simulink model "pfb_fir_8192chb_core"  (R2016b)
settings: Solver=ode45  StartTime=0.0  StopTime=10.0  RelTol=1e-3  EnableMultiTasking=on
undefined symbols (not defined in the file or in its folder): pfb_coeff_gen_calc
libraries: xbsIndex_r4 x853, casper_library_delays x48, simulink x2
(part 1 of 11)
settings Model: Creator=zaki  LastModifiedBy=kocz
settings DataIOCC: LimitDataPoints=on  SaveFormat=Array  SignalLoggingSaveFormat=ModelDataLogs
settings OptimizationCC: ExpressionDepthLimit=2147483647  LifeSpan=inf
settings DebuggingCC: UnderspecifiedInitializationDetection=Classic  MergeDetectMultiDrivingBlocksExec=none  SolverPrmCheckMsg=warning  FcnCallInpInsideContextMsg=warning  StateNameClashWarn=warning  SFUnexpectedBacktrackingDiag=warning  SFNoUnconditionalDefaultTransitionDiag=warning  SFExecutionAtInitializationDiag=none
settings HardwareCC: ProdBitPerPointer=32  ProdBitPerSizeT=32  ProdBitPerPtrDiffT=32  ProdLargestAtomicFloat=None  ProdIntDivRoundTo=Undefined  ProdEndianess=Unspecified  ProdWordSize=32  ProdHWDeviceType=32-bit Generic
settings ModelReferenceCC: PropagateSignalLabelsOutOfModel=off
settings GRTTargetCC: TargetLangStandard=C89/C90 (ANSI)  GeneratePreprocessorConditionals=Disable all  CombineOutputUpdateFcns=off  GRTInterface=on
settings ConfigComp: CovMetricSettings=dw  CovHtmlReporting=on  CovSaveCumulativeToWorkspaceVar=on  CovSaveSingleToWorkspaceVar=on  CovExternalEMLEnable=off

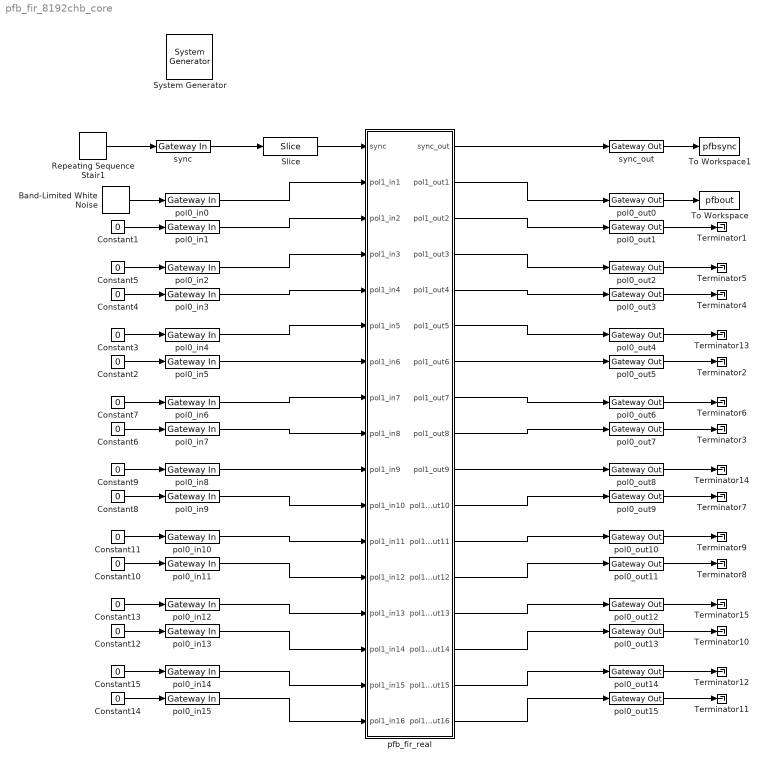
== system pfb_fir_8192chb_core ==
  " System Generator" : xbsIndex_r4/ System Generator  Tag=genX  xilinxfamily=kintex7  part=xc7k160t  speed=-2  package=ffg676  synthesis_tool=Synplify Pro  clock_wrapper=Clock Enables  directory=./pfb_fir_8192chb_core  proj_type=Project Navigator  Synth_file=XST Defaults  Impl_file=ISE Defaults  testbench=off  simulink_period=1  sysclk_period=5  dcm_input_clock_period=100  incr_netlist=off  trim_vbits=Everywhere in SubSystem  dbl_ovrd=According to Block Masks  core_generation=According to Block Masks  run_coregen=off  deprecated_control=off  eval_field=0  block_type=sysgen
      settings: block_version=10.1.3
  Band-Limited White Noise : simulink/Sources/Band-Limited White Noise  Cov=(16/128)^2  Ts=1  seed=[23341]
  Constant{1..15} (15 alike) : Constant  Value=0
  Repeating Sequence Stair1 : simulink/Sources/Repeating Sequence Stair  OutValues=[1, zeros(1,2^12-1)]  tsamp=1  OutMin=[]  OutMax=[]  OutDataTypeStr=float('double')  OutputDataTypeScalingMode=Specify via dialog  OutDataType=float('double')  ConRadixGroup=Best Precision: Vector-wise  OutScaling=2^-12
  Slice : xbsIndex_r4/Slice  nbits=3  boolean_output=on  mode=Lower Bit Location + Width  bit1=0  base1=MSB of Input  bit0=0  base0=LSB of Input  dbl_ovrd=off  block_type=slice
  Terminator{1..15} (15 alike) : Terminator
  To Workspace : ToWorkspace  VariableName=pfbout  SampleTime=-1
  To Workspace1 : ToWorkspace  VariableName=pfbsync  SampleTime=-1
  pfb_fir_real : Subsystem  Tag=casper:pfb_fir_real  AncestorBlock=casper_library_pfbs/pfb_fir_real  mask(pfb_fir_real){PFBSize=14, TotalTaps=4, WindowType=hamming, n_inputs=4, MakeBiplex=off, BitWidthIn=8, BitWidthOut=18, CoeffBitWidth=18, CoeffDistMem=off, add_latency=1, mult_latency=2, bram_latency=2, fan_latency=1, conv_latency=1, quantization=Round  (unbiased: Even Values), fwidth=1, mult_spec=2, adder_folding=on, adder_imp=DSP48, coeffs_share=off, n_pol_blocks=8}
      mask prompts: PFBSize "Size of PFB: (2^? pnts)"; TotalTaps "Total Number of Taps:"; WindowType "Windowing Function:"; n_inputs "Number of Simultaneous Inputs: (2^?)"; MakeBiplex "Make Biplex?"; BitWidthIn "Input Bitwidth:"; BitWidthOut "Output Bitwidth:"; CoeffBitWidth "Coefficient Bitwidth:"; CoeffDistMem "Use Distributed Memory for Coeffs"; add_latency "Add Latency"; mult_latency "Mult Latency"; bram_latency "BRAM Latency"; fan_latency "Fanout latency"; conv_latency "Convert latency"; quantization "Quantization Behavior"; fwidth "Bin Width Scaling (normal=1)"; mult_spec "Multiplier specification (0=core, 1=embedded, 2=behavioural) (left=1st tap, or just one value)"; adder_folding "Fold adders into DSPs"; adder_imp "Adder implementation"; coeffs_share "Share coefficients between polarisations (use less BRAM)?"; n_pol_blocks "Number of serial polarization blocks"
      mask help:
      | Fold adders into DSPs: Causes adders to be absorbed into DSP blocks (supported in Virtex5)
      | Adder implementation: Cores using Fabric or DSP48 or behavioral HDL
      mask init:
      | pfb_fir_real_init(gcb, ...
      |     'PFBSize', PFBSize, ...
      |     'TotalTaps', TotalTaps, ...
      |     'WindowType', WindowType, ...
      |     'n_inputs', n_inputs, ...
      |     'n_pol_blocks', n_pol_blocks, ...
      |     'MakeBiplex', MakeBiplex, ...
      |     'BitWidthIn', BitWidthIn, ...
      |     'BitWidthOut', BitWidthOut, ...
      |     'CoeffBitWidth', CoeffBitWidth, ...
      |     'CoeffDistMem', CoeffDistMem, ...
      |     'add_latency', add_latency, ...
      |     'mult_latency', mult_latency, ...
      |     'bram_latency', bram_latency, ...
      |     'fan_latency', fan_latency, ...
      |     'conv_latency', conv_latency, ...
      |     'quantization', quantization, ...
      |     'fwidth', fwidth, ...
      |     'mult_spec', mult_spec, ...
      |     'adder_folding', adder_folding, ...
      |     'adder_imp', adder_imp, ...
      |     'coeffs_share', coeffs_share);
      settings: AttributesFormatString=taps=4, add_latency=1
      mask Help: eval('xlWeb(''http://casper.berkeley.edu/wiki/Pfb_fir_real'')')
      mask Callback TotalTaps:
      | %num_taps = eval(get_param(gcb, 'TotalTaps'));
      | %old_vec = eval(get_param(gcb, 'mult_spec'));=-0l
      | 
      | %vec = 2.*ones(1,num_taps);
      | %old_size = length(old_vec);
      | 
      | %if(old_size <= num_taps),
      | %    new_size = old_size;
      | %else,
      | %    new_size = num_taps;
      | %end
      | 
      | %for n = 1:new_size, vec(n) = old_vec(n); end
      | %set_param(gcb, 'mult_spec', mat2str(vec));
      mask TypeOptions WindowType: bartlett | barthannwin | blackman | blackmanharris | bohamwin | chebwin | flattopwin | gausswin | hamming | hann | kaiser | nuttallwin | parzenwin | rectwin | tukeywin | triang | userwindow
      mask TypeOptions quantization: Truncate | Round  (unbiased: +/- Inf) | Round  (unbiased: Even Values)
      mask TypeOptions adder_imp: Behavioral | Fabric | DSP48
  pol0_in{0..15} (16 alike) : xbsIndex_r4/Gateway In  gui_display_data_type=Fixed-point  arith_type="Signed  (2's comp)"  n_bits=8  bin_pt=7  preci_type=Single  exp_width=8  frac_width=24  rows=1  columns=1  quantization="Round  (unbiased: +/- Inf)"  overflow=Saturate  period=1  UseAsADC=off  ADCChannel='1'  interface=None  automatic_assignment=on  address_offset=hex2dec('00')  intf_name=''  intf_description=''  default_value=0  timing_constraint=None  locs_specified=off  LOCs={}  io_standard={}  inherit_from_input=off  hdl_port=on  dbl_ovrd=off  block_type=gatewayin
      settings: infoedit="Gateway in block.  Converts inputs of type Simulink integer, double and fixed point to  Xilinx fixed point type.<P><P>Hardware notes:  In hardware these blocks become top level input ports."  block_version=10.1.3
  pol0_out{0..15} (16 alike) : xbsIndex_r4/Gateway Out  inherit_from_input=off  hdl_port=on  rows=1  columns=1  UseAsDAC=off  DACChannel='1'  interface=None  automatic_assignment=on  address_offset=hex2dec('00')  intf_name=''  intf_description=''  timing_constraint=None  locs_specified=off  LOCs={}  io_standard={}  block_type=gatewayout
      settings: infoedit="Gateway out block.  Converts Xilinx fixed point inputs into ouputs of type Simulink integer, double, or fixed point.<P><P>Hardware notes:  In hardware these blocks become top level output ports or are discarded, depending on how they are configured."  block_version=10.1.3
  sync : xbsIndex_r4/Gateway In  gui_display_data_type=Fixed-point  arith_type=Unsigned  n_bits=32  bin_pt=0  preci_type=Single  exp_width=8  frac_width=24  rows=1  columns=1  quantization="Round  (unbiased: +/- Inf)"  overflow=Saturate  period=1  UseAsADC=off  ADCChannel='1'  interface=None  automatic_assignment=on  address_offset=hex2dec('00')  intf_name=''  intf_description=''  default_value=0  timing_constraint=None  locs_specified=off  LOCs={}  io_standard={}  inherit_from_input=off  hdl_port=on  dbl_ovrd=off  block_type=gatewayin
      settings: block_version=10.1.3
  sync_out : xbsIndex_r4/Gateway Out  inherit_from_input=off  hdl_port=on  rows=1  columns=1  UseAsDAC=off  DACChannel='1'  interface=None  automatic_assignment=on  address_offset=hex2dec('00')  intf_name=''  intf_description=''  timing_constraint=None  locs_specified=off  LOCs={}  io_standard={}  block_type=gatewayout
      settings: infoedit="Gateway out block.  Converts Xilinx fixed point inputs into ouputs of type Simulink integer, double, or fixed point.<P><P>Hardware notes:  In hardware these blocks become top level output ports or are discarded, depending on how they are configured."  block_version=10.1.3
  wires:
  sync/1 -> Slice/1
  Band-Limited White Noise/1 -> pol0_in0/1
  Constant1/1 -> pol0_in1/1
  pol0_out0/1 -> To Workspace/1
  pol0_out1/1 -> Terminator1/1
  Repeating Sequence Stair1/1 -> sync/1
  sync_out/1 -> To Workspace1/1
  pfb_fir_real/1(sync_out) -> sync_out/1
  Constant5/1 -> pol0_in2/1
  Constant4/1 -> pol0_in3/1
  pol0_out2/1 -> Terminator5/1
  pol0_out3/1 -> Terminator4/1
  Slice/1 -> pfb_fir_real/1(sync)
  Constant3/1 -> pol0_in4/1
  Constant2/1 -> pol0_in5/1
  Constant7/1 -> pol0_in6/1
  Constant6/1 -> pol0_in7/1
  Constant9/1 -> pol0_in8/1
  Constant8/1 -> pol0_in9/1
  Constant11/1 -> pol0_in10/1
  Constant10/1 -> pol0_in11/1
  Constant13/1 -> pol0_in12/1
  Constant12/1 -> pol0_in13/1
  Constant15/1 -> pol0_in14/1
  Constant14/1 -> pol0_in15/1
  pol0_out4/1 -> Terminator13/1
  pol0_out5/1 -> Terminator2/1
  pol0_out6/1 -> Terminator6/1
  pol0_out7/1 -> Terminator3/1
  pol0_out8/1 -> Terminator14/1
  pol0_out9/1 -> Terminator7/1
  pol0_out10/1 -> Terminator9/1
  pol0_out11/1 -> Terminator8/1
  pol0_out12/1 -> Terminator15/1
  pol0_out13/1 -> Terminator10/1
  pol0_out14/1 -> Terminator12/1
  pol0_out15/1 -> Terminator11/1
  pol0_in1/1 -> pfb_fir_real/3(pol1_in2)
  pol0_in0/1 -> pfb_fir_real/2(pol1_in1)
  pol0_in5/1 -> pfb_fir_real/7(pol1_in6)
  pol0_in8/1 -> pfb_fir_real/10(pol1_in9)
  pol0_in7/1 -> pfb_fir_real/9(pol1_in8)
  pol0_in10/1 -> pfb_fir_real/12(pol1_in11)
  pol0_in3/1 -> pfb_fir_real/5(pol1_in4)
  pol0_in6/1 -> pfb_fir_real/8(pol1_in7)
  pol0_in9/1 -> pfb_fir_real/11(pol1_in10)
  pol0_in4/1 -> pfb_fir_real/6(pol1_in5)
  pol0_in12/1 -> pfb_fir_real/14(pol1_in13)
  pol0_in11/1 -> pfb_fir_real/13(pol1_in12)
  pol0_in14/1 -> pfb_fir_real/16(pol1_in15)
  pol0_in2/1 -> pfb_fir_real/4(pol1_in3)
  pol0_in13/1 -> pfb_fir_real/15(pol1_in14)
  pol0_in15/1 -> pfb_fir_real/17(pol1_in16)
  pfb_fir_real/7(pol1_out6) -> pol0_out5/1
  pfb_fir_real/10(pol1_out9) -> pol0_out8/1
  pfb_fir_real/5(pol1_out4) -> pol0_out3/1
  pfb_fir_real/9(pol1_out8) -> pol0_out7/1
  pfb_fir_real/12(pol1_out11) -> pol0_out10/1
  pfb_fir_real/8(pol1_out7) -> pol0_out6/1
  pfb_fir_real/3(pol1_out2) -> pol0_out1/1
  pfb_fir_real/6(pol1_out5) -> pol0_out4/1
  pfb_fir_real/14(pol1_out13) -> pol0_out12/1
  pfb_fir_real/11(pol1_out10) -> pol0_out9/1
  pfb_fir_real/13(pol1_out12) -> pol0_out11/1
  pfb_fir_real/16(pol1_out15) -> pol0_out14/1
  pfb_fir_real/4(pol1_out3) -> pol0_out2/1
  pfb_fir_real/2(pol1_out1) -> pol0_out0/1
  pfb_fir_real/15(pol1_out14) -> pol0_out13/1
  pfb_fir_real/17(pol1_out16) -> pol0_out15/1
